simulink model "Uppgift2"  (R2016a)
settings: Solver=VariableStepAuto  StartTime=0.0  StopTime=100  RelTol=1e-3
values from neighbouring files (symbols this model uses):
  C = 0.2    [Uppgift2Script.m]
  K = 1    [Uppgift2Script.m]
  M = 1    [Uppgift2Script.m]
settings Model: Creator=Samuel  LastModifiedBy=Samuel

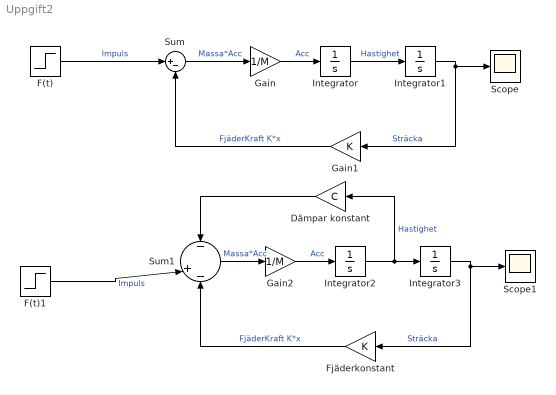
== system Uppgift2 ==
  Dämpar konstant : Gain  Gain=C
  F(t) : Step  Time=0  SampleTime=0
  F(t)1 : Step  Time=0  SampleTime=0
  Fjäderkonstant : Gain  Gain=K
  Gain : Gain  Gain=1/M
  Gain1 : Gain  Gain=K
  Gain2 : Gain  Gain=1/M
  Integrator{,1..3} (4 alike) : Integrator
  Scope : Scope
  Scope1 : Scope
  Sum : Sum  Inputs=|+-
  Sum1 : Sum  Inputs=-|+-
  wires:
  F(t)/1 -> Sum/1  "Impuls"
  Sum/1 -> Gain/1  "Massa*Acc"
  Gain/1 -> Integrator/1  "Acc"
  Integrator/1 -> Integrator1/1  "Hastighet"
  Integrator1/1 -> Scope/1, Gain1/1  "Sträcka"
  Gain1/1 -> Sum/2  "FjäderKraft K*x"
  Sum1/1 -> Gain2/1  "Massa*Acc"
  Gain2/1 -> Integrator2/1  "Acc"
  Integrator2/1 -> Dämpar konstant/1, Integrator3/1  "Hastighet"
  Integrator3/1 -> Scope1/1, Fjäderkonstant/1  "Sträcka"
  F(t)1/1 -> Sum1/2  "Impuls"
  Fjäderkonstant/1 -> Sum1/3  "FjäderKraft K*x"
  Dämpar konstant/1 -> Sum1/1
